simulink model "TPDeux"  (R2023b)
settings: Solver=VariableStepAuto  StartTime=0.0  StopTime=40  RelTol=1e-3
values from neighbouring files (symbols this model uses):
  L = 1000    [TP2.m]
libraries: slpidlib x2
settings Model: LastModifiedBy=robot
settings ModelReferenceCC: UpdateModelReferenceTargets=IfOutOfDate
settings RTWCC: GPUComputeCapability=5.0

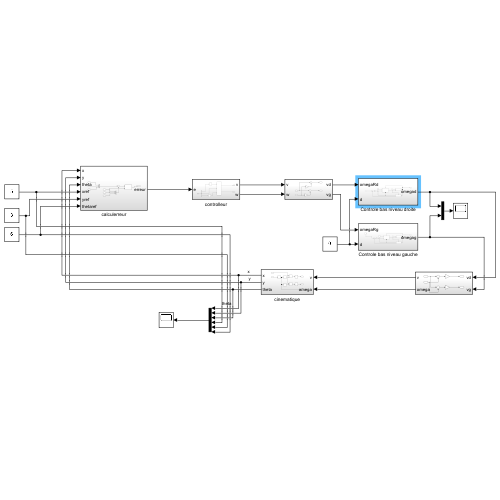
[thumbnail: Simulink's stored preview of the top-level diagram]
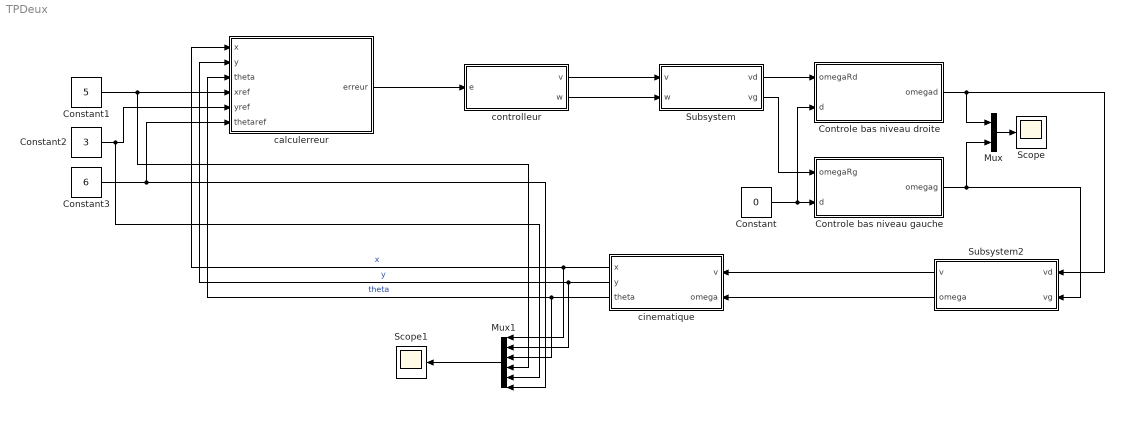
== system TPDeux ==
  Constant : Constant  Value=0
  Constant1 : Constant  Value=5
  Constant2 : Constant  Value=3
  Constant3 : Constant  Value=6
  Controle bas niveau droite : Subsystem
  Controle bas niveau gauche : Subsystem
  Mux : Mux  Inputs=2
  Mux1 : Mux  Inputs=6
  Scope : Scope
  Scope1 : Scope
  Subsystem : Subsystem
  Subsystem2 : Subsystem
  calculerreur : Subsystem
  cinematique : Subsystem
  controlleur : Subsystem
  wires:
  Subsystem/1(vd) -> Controle bas niveau droite/1(omegaRd)
  Subsystem/2(vg) -> Controle bas niveau gauche/1(omegaRg)
  Constant/1 -> Controle bas niveau droite/2(d), Controle bas niveau gauche/2(d)
  Mux/1 -> Scope/1
  Controle bas niveau droite/1(omegad) -> Mux/1, Subsystem2/1(vd)
  Controle bas niveau gauche/1(omegag) -> Mux/2, Subsystem2/2(vg)
  Subsystem2/1(v) -> cinematique/1(v)
  Subsystem2/2(omega) -> cinematique/2(omega)
  cinematique/1(x) -> calculerreur/1(x), Mux1/1  "x"
  cinematique/2(y) -> calculerreur/2(y), Mux1/2  "y"
  cinematique/3(theta) -> calculerreur/3(theta), Mux1/3  "theta"
  calculerreur/1(erreur) -> controlleur/1(e)
  Mux1/1 -> Scope1/1
  Constant1/1 -> Mux1/4, calculerreur/4(xref)
  Constant2/1 -> Mux1/5, calculerreur/5(yref)
  Constant3/1 -> Mux1/6, calculerreur/6(thetaref)
  controlleur/1(v) -> Subsystem/1(v)
  controlleur/2(w) -> Subsystem/2(w)

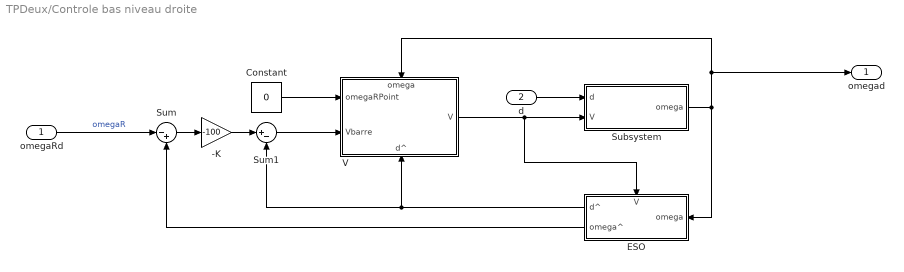
== system TPDeux/Controle bas niveau droite ==
  omegaRd : Inport
  d : Inport  Port=2
  -K : Gain  Gain=-100
  Constant : Constant  Value=0
  ESO : Subsystem
      settings: PortSchema="{\"entries\":[{\"content\":{\"sides\":[{\"content\":{\"connectorIds\":[\"In1\"]},\"type\":\"ConnectorPlacement.EquallySpacedRectSide\",\"uuid\":\"e1c274ad-ba20-48aa-bf77-d813922b9d8c\"},{\"content\":{\"connectorIds\":[\"Out1\",\"Out2\"],\"side\":\"RIGHT\"},\"type\":\"ConnectorPlacement.EquallySpacedRectSide\",\"uuid\":\"e0452d8d-59d0-4149-8f5d-8992181ff20f\"},{\"content\":{\"connectorIds\":[\"In2\"],\"side\":\"TOP\"},\"type\":\"ConnectorPlacement.EquallySpacedRectSide\",\"uuid\":\"2555fc7c-6481-4291-bd13-a8877dfa9dc8\"}]},\"type\":\"ConnectorPlacement.EquallySpacedConnector\",\"uuid\":\"299a756b-03db-4de2-a07a-503eb175a86e\"}],\"packageUris\":[\"http://schema.mathworks.com/mf0/Connector/R2020b\"],\"version\":\"1.0\"}"
  Subsystem : Subsystem
  Sum : Sum  Inputs=|-+
  Sum1 : Sum  Inputs=|+-
  V : Subsystem
      settings: PortSchema="{\"entries\":[{\"content\":{\"sides\":[{\"content\":{\"connectorIds\":[\"In1\",\"In2\"]},\"type\":\"ConnectorPlacement.EquallySpacedRectSide\",\"uuid\":\"3806cb88-ac27-4e54-9602-5c269981dd4a\"},{\"content\":{\"connectorIds\":[\"Out1\"],\"side\":\"RIGHT\"},\"type\":\"ConnectorPlacement.EquallySpacedRectSide\",\"uuid\":\"4ee9a9f2-7c78-4ee8-8e7a-01ce00e7f290\"},{\"content\":{\"connectorIds\":[\"In3\"],\"side\":\"TOP\"},\"type\":\"ConnectorPlacement.EquallySpacedRectSide\",\"uuid\":\"e264f9c5-56fc-47fc-809a-fa74c803b869\"},{\"content\":{\"connectorIds\":[\"In4\"],\"side\":\"BOTTOM\"},\"type\":\"ConnectorPlacement.EquallySpacedRectSide\",\"uuid\":\"4158efb2-b17f-4939-9c93-ac5329091cca\"}]},\"type\":\"ConnectorPlacement.EquallySpacedConnector\",\"uuid\":\"47b4022f-b71e-4683-9257-d4ec3ed1dae1\"}],\"packageUris\":[\"http://schema.mathworks.com/mf0/Connector/R2020b\"],\"version\":\"1.0\"}"
  omegad : Outport
  wires:
  ESO/2(omega^) -> Sum/2
  Subsystem/1(omega) -> ESO/1(omega), V/3(omega), omegad/1
  ESO/1(d^) -> V/4(d^), Sum1/2
  V/1(V) -> ESO/2(V), Subsystem/2(V)
  Sum/1 -> -K/1
  Sum1/1 -> V/2(Vbarre)
  -K/1 -> Sum1/1
  omegaRd/1 -> Sum/1  "omegaR"
  d/1 -> Subsystem/1(d)
  Constant/1 -> V/1(omegaRPoint)

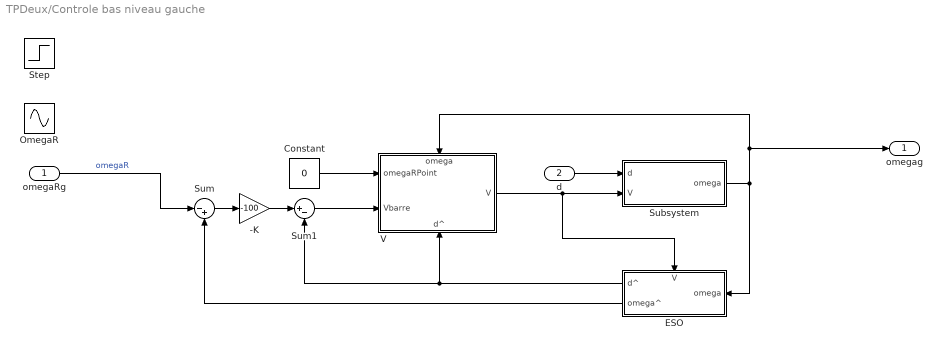
== system TPDeux/Controle bas niveau gauche ==
  omegaRg : Inport
  d : Inport  Port=2
  -K : Gain  Gain=-100
  Constant : Constant  Value=0
  ESO : Subsystem
      settings: PortSchema="{\"entries\":[{\"content\":{\"sides\":[{\"content\":{\"connectorIds\":[\"In1\"]},\"type\":\"ConnectorPlacement.EquallySpacedRectSide\",\"uuid\":\"e1c274ad-ba20-48aa-bf77-d813922b9d8c\"},{\"content\":{\"connectorIds\":[\"Out1\",\"Out2\"],\"side\":\"RIGHT\"},\"type\":\"ConnectorPlacement.EquallySpacedRectSide\",\"uuid\":\"e0452d8d-59d0-4149-8f5d-8992181ff20f\"},{\"content\":{\"connectorIds\":[\"In2\"],\"side\":\"TOP\"},\"type\":\"ConnectorPlacement.EquallySpacedRectSide\",\"uuid\":\"2555fc7c-6481-4291-bd13-a8877dfa9dc8\"}]},\"type\":\"ConnectorPlacement.EquallySpacedConnector\",\"uuid\":\"299a756b-03db-4de2-a07a-503eb175a86e\"}],\"packageUris\":[\"http://schema.mathworks.com/mf0/Connector/R2020b\"],\"version\":\"1.0\"}"
  OmegaR : Sin  Amplitude=2  Bias=4  Frequency=0.5  SampleTime=0
  Step : Step  Time=3  After=2  SampleTime=0
  Subsystem : Subsystem
  Sum : Sum  Inputs=|-+
  Sum1 : Sum  Inputs=|+-
  V : Subsystem
      settings: PortSchema="{\"entries\":[{\"content\":{\"sides\":[{\"content\":{\"connectorIds\":[\"In1\",\"In2\"]},\"type\":\"ConnectorPlacement.EquallySpacedRectSide\",\"uuid\":\"3806cb88-ac27-4e54-9602-5c269981dd4a\"},{\"content\":{\"connectorIds\":[\"Out1\"],\"side\":\"RIGHT\"},\"type\":\"ConnectorPlacement.EquallySpacedRectSide\",\"uuid\":\"4ee9a9f2-7c78-4ee8-8e7a-01ce00e7f290\"},{\"content\":{\"connectorIds\":[\"In3\"],\"side\":\"TOP\"},\"type\":\"ConnectorPlacement.EquallySpacedRectSide\",\"uuid\":\"e264f9c5-56fc-47fc-809a-fa74c803b869\"},{\"content\":{\"connectorIds\":[\"In4\"],\"side\":\"BOTTOM\"},\"type\":\"ConnectorPlacement.EquallySpacedRectSide\",\"uuid\":\"4158efb2-b17f-4939-9c93-ac5329091cca\"}]},\"type\":\"ConnectorPlacement.EquallySpacedConnector\",\"uuid\":\"47b4022f-b71e-4683-9257-d4ec3ed1dae1\"}],\"packageUris\":[\"http://schema.mathworks.com/mf0/Connector/R2020b\"],\"version\":\"1.0\"}"
  omegag : Outport
  wires:
  ESO/2(omega^) -> Sum/2
  Subsystem/1(omega) -> ESO/1(omega), V/3(omega), omegag/1
  ESO/1(d^) -> V/4(d^), Sum1/2
  V/1(V) -> ESO/2(V), Subsystem/2(V)
  Sum/1 -> -K/1
  Sum1/1 -> V/2(Vbarre)
  -K/1 -> Sum1/1
  omegaRg/1 -> Sum/1  "omegaR"
  d/1 -> Subsystem/1(d)
  Constant/1 -> V/1(omegaRPoint)

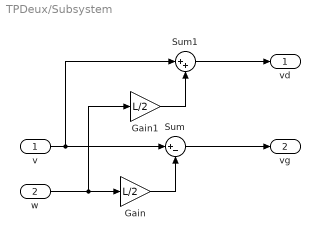
== system TPDeux/Subsystem ==
  v : Inport
  w : Inport  Port=2
  Gain : Gain  Gain=L/2
  Gain1 : Gain  Gain=L/2
  Sum : Sum  Inputs=|+-
  Sum1 : Sum  Inputs=|++
  vd : Outport
  vg : Outport  Port=2
  wires:
  w/1 -> Gain1/1, Gain/1
  Gain/1 -> Sum/2
  v/1 -> Sum1/1, Sum/1
  Sum/1 -> vg/1
  Gain1/1 -> Sum1/2
  Sum1/1 -> vd/1

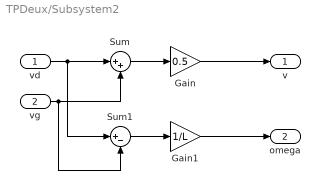
== system TPDeux/Subsystem2 ==
  vd : Inport
  vg : Inport  Port=2
  Gain : Gain  Gain=0.5
  Gain1 : Gain  Gain=1/L
  Sum : Sum  Inputs=|++
  Sum1 : Sum  Inputs=|+-
  v : Outport
  omega : Outport  Port=2
  wires:
  vd/1 -> Sum1/1, Sum/1
  vg/1 -> Sum1/2, Sum/2
  Sum/1 -> Gain/1
  Gain/1 -> v/1
  Sum1/1 -> Gain1/1
  Gain1/1 -> omega/1

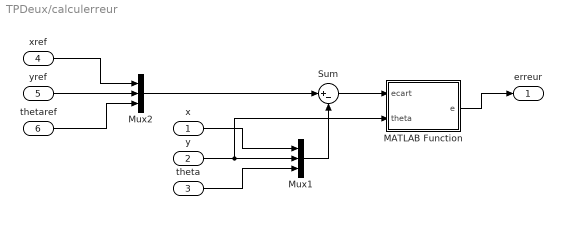
== system TPDeux/calculerreur ==
  x : Inport
  y : Inport  Port=2
  theta : Inport  Port=3
  xref : Inport  Port=4
  yref : Inport  Port=5
  thetaref : Inport  Port=6
  MATLAB Function : MATLAB Function  TreatAsAtomicUnit=on
  Mux1 : Mux  Inputs=3
  Mux2 : Mux  Inputs=3
  Sum : Sum  Inputs=|+-
  erreur : Outport
  wires:
  theta/1 -> Mux1/3
  yref/1 -> Mux2/2
  xref/1 -> Mux2/1
  thetaref/1 -> Mux2/3
  Mux2/1 -> Sum/1
  y/1 -> MATLAB Function/2(theta), Mux1/2
  Mux1/1 -> Sum/2
  x/1 -> Mux1/1
  Sum/1 -> MATLAB Function/1(ecart)
  MATLAB Function/1(e) -> erreur/1

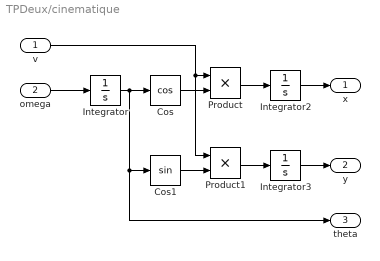
== system TPDeux/cinematique ==
  v : Inport
  omega : Inport  Port=2
  Cos : Trigonometry  Operator=cos
  Cos1 : Trigonometry
  Integrator : Integrator
  Integrator2 : Integrator
  Integrator3 : Integrator
  Product : Product
  Product1 : Product
  x : Outport
  y : Outport  Port=2
  theta : Outport  Port=3
  wires:
  v/1 -> Product1/1, Product/1
  Cos/1 -> Product/2
  omega/1 -> Integrator/1
  Integrator/1 -> theta/1, Cos1/1, Cos/1
  Cos1/1 -> Product1/2
  Product/1 -> Integrator2/1
  Product1/1 -> Integrator3/1
  Integrator2/1 -> x/1
  Integrator3/1 -> y/1

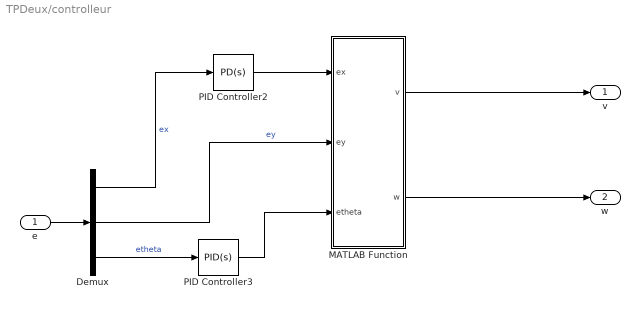
== system TPDeux/controlleur ==
  e : Inport
  Demux : Demux  Outputs=3
  MATLAB Function : MATLAB Function  TreatAsAtomicUnit=on
  PID Controller2 : slpidlib/PID Controller  Controller=PD  Form=Parallel  TimeDomain=Continuous-time  UseExternalTs=off  SampleTime=-1  IntegratorMethod=Forward Euler  FilterMethod=Forward Euler  ControllerParametersSource=internal  P=1  I=1  UseKiTs=off  D=1  N=100  UseFilter=on  TunerSelectOption=Transfer Function Based (PID Tuner App)  InitialConditionSource=internal  InitialConditionForIntegrator=0  InitialConditionForFilter=0  DifferentiatorICPrevScaledInput=0  ExternalReset=none  TrackingMode=off  Kt=1  LimitOutput=off  SatLimitsSource=internal  UpperSaturationLimit=inf  LowerSaturationLimit=-inf  LinearizeAsGain=on  AntiWindupMode=none  Kb=1  LimitIntegrator=off  UpperIntegratorSaturationLimit=inf  LowerIntegratorSaturationLimit=-inf  POutMin=[]  POutMax=[]  IOutMin=[]  IOutMax=[]  DOutMin=[]  DOutMax=[]  NOutMin=[]  NOutMax=[]  SumOutMin=[]  SumOutMax=[]  SaturationOutMin=[]  SaturationOutMax=[]  PParamMin=[]  PParamMax=[]  IParamMin=[]  IParamMax=[]  DParamMin=[]  DParamMax=[]  NParamMin=[]  NParamMax=[]  KbParamMin=[]  KbParamMax=[]  KtParamMin=[]  KtParamMax=[]  KbOutMin=[]  KbOutMax=[]  KtOutMin=[]  KtOutMax=[]  IntegratorOutMin=[]  IntegratorOutMax=[]  FilterOutMin=[]  FilterOutMax=[]  SumI1OutMin=[]  SumI1OutMax=[]  SumI2OutMin=[]  SumI2OutMax=[]  SumI3OutMin=[]  SumI3OutMax=[]  SumI4OutMin=[]  SumI4OutMax=[]  SumDOutMin=[]  SumDOutMax=[]  DifferentiatorOutMin=[]  DifferentiatorOutMax=[]  FilterDiffOutCoefMin=[]  FilterDiffOutCoefMax=[]  ReciprocalOutMin=[]  ReciprocalOutMax=[]  SumDenOutMin=[]  SumDenOutMax=[]  SumNumOutMin=[]  SumNumOutMax=[]  DivideOutMin=[]  DivideOutMax=[]  UdiffTsProdOutMin=[]  UdiffTsProdOutMax=[]  NTsProdOutMin=[]  NTsProdOutMax=[]  UintegralTsProdOutMin=[]  UintegralTsProdOutMax=[]  UngainTsProdOutMin=[]  UngainTsProdOutMax=[]  ClampingZeroOutDataTypeStr=Inherit: Inherit via back propagation  ClampingZeroOutMin=[]  ClampingZeroOutMax=[]  FilterDenConstantOutDataTypeStr=Inherit: Inherit via back propagation  FilterDenConstantOutMin=[]  FilterDenConstantOutMax=[]  PCopyOutDataTypeStr=Inherit: Inherit via back propagation  PCopyOutMin=[]  PCopyOutMax=[]  NCopyOutDataTypeStr=Inherit: Inherit via back propagation  NCopyOutMin=[]  NCopyOutMax=[]  IntegratorContinuousStateAttributes=''  IntegratorStateMustResolveToSignalObject=off  IntegratorRTWStateStorageClass=Auto  FilterContinuousStateAttributes=''  FilterStateMustResolveToSignalObject=off  FilterRTWStateStorageClass=Auto  ParallelPVariant=InternalParameters  IdealPVariant=Disabled  IVariant=Disabled  DVariant=InternalParameters  IntegratorVariant=Disabled  SatVariant=Disabled  AWVariant=Disabled  PCopyVariant=Disabled  TRVariant=Disabled  FdbkBlocksVariant=Forward  IdealPFdbkVariant=Disabled  SatFdbkVariant=Disabled  DerivativeFilterVariant=ContFilter  NVariant=InternalParameters  NCopyVariant=Disabled  FilterICVariant=InternalICsFilter  IntegratorICVariant=Disabled  ExternalResetVariant=Disabled  TRSumVariant=Passthrough  SumFdbkVariant=Disabled  SumVariant=Sum_PD  TsampFilterVariant=InternalTs  TsampNgainVariant=Passthrough  TsampIntegralVariant=Disabled_SignalSpec  ExternalSaturationOutDataTypeStr=Inherit: Same as second input
  PID Controller3 : slpidlib/PID Controller  Controller=PID  Form=Parallel  TimeDomain=Continuous-time  UseExternalTs=off  SampleTime=-1  IntegratorMethod=Forward Euler  FilterMethod=Forward Euler  ControllerParametersSource=internal  P=1  I=1  UseKiTs=off  D=1  N=100  UseFilter=on  TunerSelectOption=Transfer Function Based (PID Tuner App)  InitialConditionSource=internal  InitialConditionForIntegrator=0  InitialConditionForFilter=0  DifferentiatorICPrevScaledInput=0  ExternalReset=none  TrackingMode=off  Kt=1  LimitOutput=off  SatLimitsSource=internal  UpperSaturationLimit=inf  LowerSaturationLimit=-inf  LinearizeAsGain=on  AntiWindupMode=none  Kb=1  LimitIntegrator=off  UpperIntegratorSaturationLimit=inf  LowerIntegratorSaturationLimit=-inf  POutMin=[]  POutMax=[]  IOutMin=[]  IOutMax=[]  DOutMin=[]  DOutMax=[]  NOutMin=[]  NOutMax=[]  SumOutMin=[]  SumOutMax=[]  SaturationOutMin=[]  SaturationOutMax=[]  PParamMin=[]  PParamMax=[]  IParamMin=[]  IParamMax=[]  DParamMin=[]  DParamMax=[]  NParamMin=[]  NParamMax=[]  KbParamMin=[]  KbParamMax=[]  KtParamMin=[]  KtParamMax=[]  KbOutMin=[]  KbOutMax=[]  KtOutMin=[]  KtOutMax=[]  IntegratorOutMin=[]  IntegratorOutMax=[]  FilterOutMin=[]  FilterOutMax=[]  SumI1OutMin=[]  SumI1OutMax=[]  SumI2OutMin=[]  SumI2OutMax=[]  SumI3OutMin=[]  SumI3OutMax=[]  SumI4OutMin=[]  SumI4OutMax=[]  SumDOutMin=[]  SumDOutMax=[]  DifferentiatorOutMin=[]  DifferentiatorOutMax=[]  FilterDiffOutCoefMin=[]  FilterDiffOutCoefMax=[]  ReciprocalOutMin=[]  ReciprocalOutMax=[]  SumDenOutMin=[]  SumDenOutMax=[]  SumNumOutMin=[]  SumNumOutMax=[]  DivideOutMin=[]  DivideOutMax=[]  UdiffTsProdOutMin=[]  UdiffTsProdOutMax=[]  NTsProdOutMin=[]  NTsProdOutMax=[]  UintegralTsProdOutMin=[]  UintegralTsProdOutMax=[]  UngainTsProdOutMin=[]  UngainTsProdOutMax=[]  ClampingZeroOutDataTypeStr=Inherit: Inherit via back propagation  ClampingZeroOutMin=[]  ClampingZeroOutMax=[]  FilterDenConstantOutDataTypeStr=Inherit: Inherit via back propagation  FilterDenConstantOutMin=[]  FilterDenConstantOutMax=[]  PCopyOutDataTypeStr=Inherit: Inherit via back propagation  PCopyOutMin=[]  PCopyOutMax=[]  NCopyOutDataTypeStr=Inherit: Inherit via back propagation  NCopyOutMin=[]  NCopyOutMax=[]  IntegratorContinuousStateAttributes=''  IntegratorStateMustResolveToSignalObject=off  IntegratorRTWStateStorageClass=Auto  FilterContinuousStateAttributes=''  FilterStateMustResolveToSignalObject=off  FilterRTWStateStorageClass=Auto  ParallelPVariant=InternalParameters  IdealPVariant=Disabled  IVariant=InternalParameters  DVariant=InternalParameters  IntegratorVariant=Continuous  SatVariant=Disabled  AWVariant=Passthrough  PCopyVariant=Disabled  TRVariant=Disabled  FdbkBlocksVariant=Forward  IdealPFdbkVariant=Disabled  SatFdbkVariant=Disabled  DerivativeFilterVariant=ContFilter  NVariant=InternalParameters  NCopyVariant=Disabled  FilterICVariant=InternalICsFilter  IntegratorICVariant=InternalICs  ExternalResetVariant=Disabled  TRSumVariant=Passthrough  SumFdbkVariant=Disabled  SumVariant=Sum_PID  TsampFilterVariant=InternalTs  TsampNgainVariant=Passthrough  TsampIntegralVariant=Disabled_SignalSpec  ExternalSaturationOutDataTypeStr=Inherit: Same as second input
  v : Outport
  w : Outport  Port=2
  wires:
  e/1 -> Demux/1
  Demux/1 -> PID Controller2/1  "ex"
  Demux/2 -> MATLAB Function/2(ey)  "ey"
  Demux/3 -> PID Controller3/1  "etheta"
  MATLAB Function/1(v) -> v/1
  MATLAB Function/2(w) -> w/1
  PID Controller2/1 -> MATLAB Function/1(ex)
  PID Controller3/1 -> MATLAB Function/3(etheta)

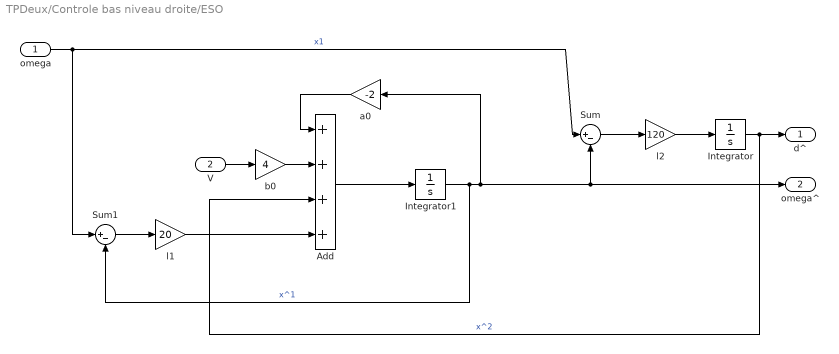
== system TPDeux/Controle bas niveau droite/ESO ==
  omega : Inport
  V : Inport  Port=2
  Add : Sum  Inputs=++++
  Integrator : Integrator
  Integrator1 : Integrator
  Sum : Sum  Inputs=|+-
  Sum1 : Sum  Inputs=|+-
  a0 : Gain  Gain=-2
  b0 : Gain  Gain=4
  l1 : Gain  Gain=20
  l2 : Gain  Gain=120
  d^ : Outport
  omega^ : Outport  Port=2
  wires:
  Integrator/1 -> Add/3, d^/1  "x^2"
  l2/1 -> Integrator/1
  Sum/1 -> l2/1
  omega/1 -> Sum/1, Sum1/1  "x1"
  Integrator1/1 -> omega^/1, Sum/2, a0/1, Sum1/2  "x^1"
  Add/1 -> Integrator1/1
  a0/1 -> Add/1
  V/1 -> b0/1
  b0/1 -> Add/2
  l1/1 -> Add/4
  Sum1/1 -> l1/1

== system TPDeux/Controle bas niveau droite/Subsystem ==
  d : Inport
  V : Inport  Port=2
  Add : Sum  Inputs=+++
  Integrator : Integrator
  a0 : Gain  Gain=-2
  b0 : Gain  Gain=4
  omega : Outport
  wires:
  d/1 -> Add/1
  a0/1 -> Add/3
  Integrator/1 -> a0/1, omega/1
  Add/1 -> Integrator/1
  V/1 -> b0/1
  b0/1 -> Add/2

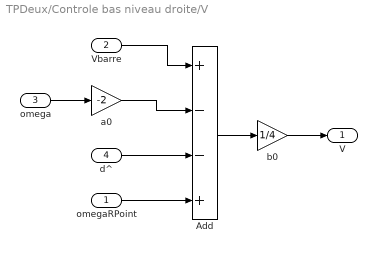
== system TPDeux/Controle bas niveau droite/V ==
  omegaRPoint : Inport
  Vbarre : Inport  Port=2
  omega : Inport  Port=3
  d^ : Inport  Port=4
  Add : Sum  Inputs=+--+
  a0 : Gain  Gain=-2
  b0 : Gain  Gain=1/4
  V : Outport
  wires:
  omega/1 -> a0/1
  Vbarre/1 -> Add/1
  Add/1 -> b0/1
  a0/1 -> Add/2
  omegaRPoint/1 -> Add/4
  d^/1 -> Add/3
  b0/1 -> V/1

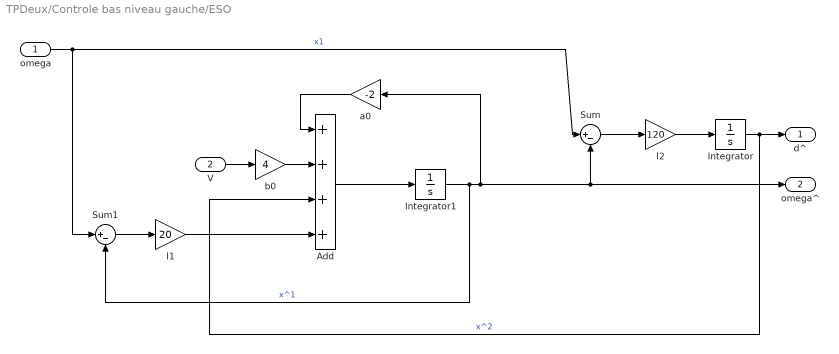
== system TPDeux/Controle bas niveau gauche/ESO ==
  omega : Inport
  V : Inport  Port=2
  Add : Sum  Inputs=++++
  Integrator : Integrator
  Integrator1 : Integrator
  Sum : Sum  Inputs=|+-
  Sum1 : Sum  Inputs=|+-
  a0 : Gain  Gain=-2
  b0 : Gain  Gain=4
  l1 : Gain  Gain=20
  l2 : Gain  Gain=120
  d^ : Outport
  omega^ : Outport  Port=2
  wires:
  Integrator/1 -> Add/3, d^/1  "x^2"
  l2/1 -> Integrator/1
  Sum/1 -> l2/1
  omega/1 -> Sum/1, Sum1/1  "x1"
  Integrator1/1 -> omega^/1, Sum/2, a0/1, Sum1/2  "x^1"
  Add/1 -> Integrator1/1
  a0/1 -> Add/1
  V/1 -> b0/1
  b0/1 -> Add/2
  l1/1 -> Add/4
  Sum1/1 -> l1/1

== system TPDeux/Controle bas niveau gauche/Subsystem ==
  d : Inport
  V : Inport  Port=2
  Add : Sum  Inputs=+++
  Integrator : Integrator
  a0 : Gain  Gain=-2
  b0 : Gain  Gain=4
  omega : Outport
  wires:
  d/1 -> Add/1
  a0/1 -> Add/3
  Integrator/1 -> a0/1, omega/1
  Add/1 -> Integrator/1
  V/1 -> b0/1
  b0/1 -> Add/2

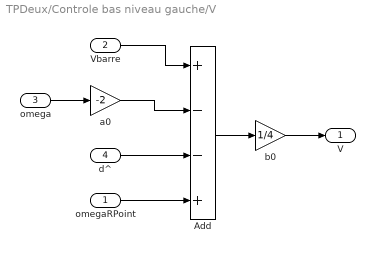
== system TPDeux/Controle bas niveau gauche/V ==
  omegaRPoint : Inport
  Vbarre : Inport  Port=2
  omega : Inport  Port=3
  d^ : Inport  Port=4
  Add : Sum  Inputs=+--+
  a0 : Gain  Gain=-2
  b0 : Gain  Gain=1/4
  V : Outport
  wires:
  omega/1 -> a0/1
  Vbarre/1 -> Add/1
  Add/1 -> b0/1
  a0/1 -> Add/2
  omegaRPoint/1 -> Add/4
  d^/1 -> Add/3
  b0/1 -> V/1

== matlab function TPDeux/controlleur/MATLAB Function ==
  data: ex input; v output; ey input; etheta input; w output
function [v,w] = fcn(ex, ey, etheta)
vr = 0;
wr = 0;
ky = 2;

v = vr*cos(etheta) + ex;
w = wr + etheta + vr*ky*ey;

== matlab function TPDeux/calculerreur/MATLAB Function ==
  data: ecart input; e output; theta input
function e = fcn(ecart, theta)

rotation_matrix = [
    cos(theta) sin(theta) 0;
    -sin(theta) cos(theta) 0
     0 0 1
    ];
e = rotation_matrix*ecart;
